simulink model "Taller_1"  (R2025b)
settings: Solver=VariableStepAuto  StartTime=0.0  StopTime=3  RelTol=1e-3
libraries: simulink x8
settings Model: Creator=andre  LastModifiedBy=andre

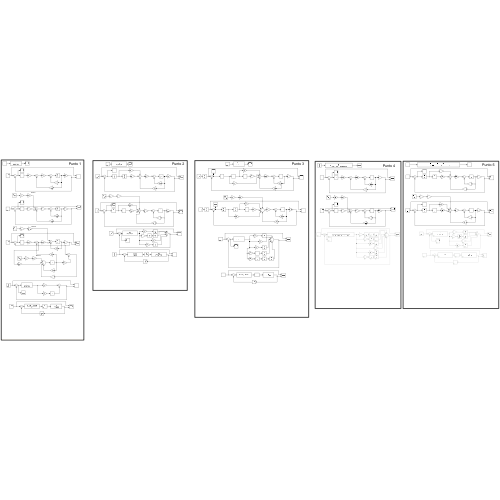
[thumbnail: Simulink's stored preview of the top-level diagram]
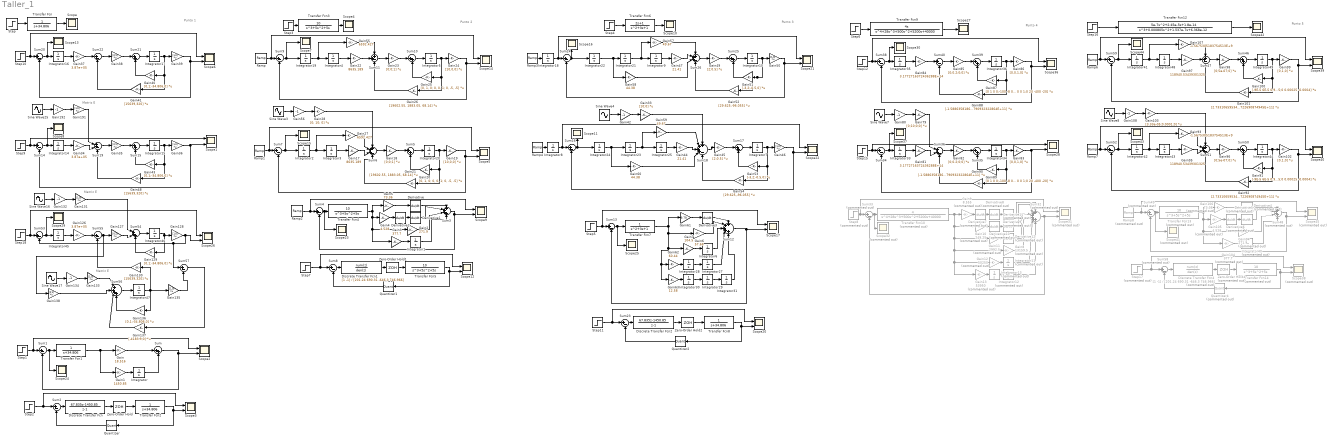
== system Taller_1 ==
  note: Punto 1
  note: Matriz E
  note: Matriz E
  note: Matriz E
  note: Punto 2
  note: Punto 3
  note: Punto 4
  note: Punto 5
  Derivative{,1..3} (4 alike) : Derivative
  Derivative{4..12} (9 alike) : Derivative  Commented=on
  Discrete Transfer Fcn : DiscreteTransferFcn  Numerator=[67.835 -1450.85]  Denominator=[1 -1]
  Discrete Transfer Fcn1 : DiscreteTransferFcn  Numerator=[1 -1]  Denominator=[201.24 690.31 -646.3 746.966]
  Discrete Transfer Fcn2 : DiscreteTransferFcn  Numerator=[67.835 -1450.85]  Denominator=[1 -1]
  Discrete Transfer Fcn4 : DiscreteTransferFcn  Commented=on  Numerator=[1 -1]  Denominator=[201.24 690.31 -646.3 746.966]
  Gain : Gain  Gain=18.516
  Gain1 : Gain  Gain=1450.85
  Gain10 : Gain  Commented=on  Gain=249.25
  Gain100 : Gain  Gain=[-9E-5 6E-5 0;9E-5 -0.000315 0.000125;0 0.00025 -0.0004]  Multiplication=Matrix(K*u)
  Gain101 : Gain  Gain=[2.7331065953402523E+13 282834.44444416161 -2.8927722690874945E+11]  Multiplication=Matrix(K*u)
  Gain102 : Gain  Gain=[0,1,0]  Multiplication=Matrix(K*u)
  Gain103 : Gain  Gain=[3.33e-05;0.0001;0]  Multiplication=Matrix(K*u)
  Gain104 : Gain  Commented=on  Gain=377.7
  Gain105 : Gain  Commented=on  Gain=4.528
  Gain106 : Gain  Commented=on  Gain=73.36
  Gain107 : Gain  Gain=-1.5675305183754513E+9
  Gain{42,56,80,108,132,134,192} (7 alike) : Gain  Gain=-1
  Gain11 : Gain  Commented=on  Gain=2992.5
  Gain12 : Gain  Commented=on  Gain=50250
  Gain126 : Gain  Gain=3.87e+05
  Gain{35,38,127,138} (4 alike) : Gain  Gain=[0;1]  Multiplication=Matrix(K*u)
  Gain{36,39,46,50,128,135} (6 alike) : Gain  Gain=[1,0]  Multiplication=Matrix(K*u)
  Gain{40,43,129,136} (4 alike) : Gain  Gain=[0,1;-34.806,0]  Multiplication=Matrix(K*u)
  Gain13 : Gain  Commented=on  Gain=53950
  Gain130 : Gain  Gain=[15639,320]  Multiplication=Matrix(K*u)
  Gain131 : Gain  Gain=[1;0]  Multiplication=Matrix(K*u)
  Gain133 : Gain  Gain=[1;0]  Multiplication=Matrix(K*u)
  Gain137 : Gain  Gain=[-4183.9;0]  Multiplication=Matrix(K*u)
  Gain17 : Gain  Gain=8635.189
  Gain18 : Gain  Gain=[0;0;1]  Multiplication=Matrix(K*u)
  Gain19 : Gain  Gain=[10,0,0]  Multiplication=Matrix(K*u)
  Gain191 : Gain  Gain=[1;0]  Multiplication=Matrix(K*u)
  Gain2 : Gain  Gain=271.9
  Gain20 : Gain  Gain=[0, 1, 0; 0, 0, 1; 0, -5, -5]  Multiplication=Matrix(K*u)
  Gain21 : Gain  Gain=[19602.55, 1883.05, 68.14]  Multiplication=Matrix(K*u)
  Gain22 : Gain  Gain=8635.189
  Gain23 : Gain  Gain=[0;0;1]  Multiplication=Matrix(K*u)
  Gain24 : Gain  Gain=[10,0,0]  Multiplication=Matrix(K*u)
  Gain25 : Gain  Gain=[0, 1, 0; 0, 0, 1; 0, -5, -5]  Multiplication=Matrix(K*u)
  Gain26 : Gain  Gain=[19602.55, 1883.05, 68.14]  Multiplication=Matrix(K*u)
  Gain27 : Gain  Gain=6592.427
  Gain28 : Gain  Gain=[0; 10; 0]  Multiplication=Matrix(K*u)
  Gain3 : Gain  Gain=377.7
  Gain33 : Gain  Gain=[10;0]  Multiplication=Matrix(K*u)
  Gain34 : Gain  Gain=3.87e+05
  Gain37 : Gain  Gain=3.87e+05
  Gain4 : Gain  Gain=4.528
  Gain41 : Gain  Gain=[15639,320]  Multiplication=Matrix(K*u)
  Gain44 : Gain  Gain=21.41
  Gain45 : Gain  Gain=[2;0.5]  Multiplication=Matrix(K*u)
  Gain47 : Gain  Gain=21.41
  Gain48 : Gain  Gain=[15639,320]  Multiplication=Matrix(K*u)
  Gain49 : Gain  Gain=[2;0.5]  Multiplication=Matrix(K*u)
  Gain5 : Gain  Gain=73.36
  Gain51 : Gain  Gain=[-3,2;-0.5,0]  Multiplication=Matrix(K*u)
  Gain52 : Gain  Gain=[29.625,-96.055]  Multiplication=Matrix(K*u)
  Gain53 : Gain  Gain=[-3,2;-0.5,0]  Multiplication=Matrix(K*u)
  Gain54 : Gain  Gain=[29.625,-96.055]  Multiplication=Matrix(K*u)
  Gain55 : Gain  Gain=6592.427
  Gain57 : Gain  Gain=49.67
  Gain58 : Gain  Gain=44.38
  Gain59 : Gain  Gain=49.67
  Gain6 : Gain  Gain=57.68
  Gain60 : Gain  Gain=44.38
  Gain61 : Gain  Gain=9.79
  Gain62 : Gain  Gain=60.44
  Gain63 : Gain  Gain=12.58
  Gain7 : Gain  Gain=104.5
  Gain79 : Gain  Gain=[0;10;0;0]  Multiplication=Matrix(K*u)
  Gain8 : Gain  Commented=on  Gain=13159.5
  Gain81 : Gain  Gain=3.1772716372436288E+14
  Gain82 : Gain  Gain=[0;0.2;0;0]  Multiplication=Matrix(K*u)
  Gain83 : Gain  Gain=[0,0,1,0]  Multiplication=Matrix(K*u)
  Gain84 : Gain  Gain=3.1772716372436288E+14
  Gain85 : Gain  Gain=[0;0.2;0;0]  Multiplication=Matrix(K*u)
  Gain86 : Gain  Gain=[0,0,1,0]  Multiplication=Matrix(K*u)
  Gain87 : Gain  Gain=[0 1 0 0;-100 -8 0 8;0 0 0 1;0 20 -400 -20]  Multiplication=Matrix(K*u)
  Gain88 : Gain  Gain=[-1.5886358186321061E+13 67.6956684856248 1.5886358185456043E+13 7.9431790932322864E+11]  Multiplication=Matrix(K*u)
  Gain89 : Gain  Gain=[0 1 0 0;-100 -8 0 8;0 0 0 1;0 20 -400 -20]  Multiplication=Matrix(K*u)
  Gain9 : Gain  Commented=on  Gain=8.555
  Gain90 : Gain  Gain=[-1.5886358186321061E+13 67.6956684856248 1.5886358185456043E+13 7.9431790932322864E+11]  Multiplication=Matrix(K*u)
  Gain91 : Gain  Gain=[-9E-5 6E-5 0;9E-5 -0.000315 0.000125;0 0.00025 -0.0004]  Multiplication=Matrix(K*u)
  Gain92 : Gain  Gain=[2.7331065953402523E+13 282834.44444416161 -2.8927722690874945E+11]  Multiplication=Matrix(K*u)
  Gain93 : Gain  Gain=-1.5675305183754513E+9
  Gain94 : Gain  Commented=on  Gain=271.9
  Gain95 : Gain  Gain=118940.53439301325
  Gain96 : Gain  Gain=[0;5e-07;0]  Multiplication=Matrix(K*u)
  Gain97 : Gain  Gain=118940.53439301325
  Gain98 : Gain  Gain=[0;5e-07;0]  Multiplication=Matrix(K*u)
  Gain99 : Gain  Gain=[0,1,0]  Multiplication=Matrix(K*u)
  Integrator{,1..10,14..25,27..31,33..36,41..49} (41 alike) : Integrator
  Integrator{11..13,40} (4 alike) : Integrator  Commented=on
  Quantizer : Quantizer  QuantizationInterval=3.3/1024
  Quantizer1 : Quantizer  QuantizationInterval=3.3/1024
  Quantizer2 : Quantizer  QuantizationInterval=3.3/1024
  Quantizer4 : Quantizer  Commented=on  QuantizationInterval=3.3/1024
  Ramp{,1..4,6..7} (7 alike) : simulink/Sources/Ramp  slope=1  start=0  InitialOutput=0
  Ramp8 : simulink/Sources/Ramp  Commented=on  slope=1  start=0  InitialOutput=0
  Scope{,4,7..8,10..11,13,15..16,23..25,27,29..30,37,42..44} (19 alike) : Scope
      Scope settings: ActiveDisplayYMinimum=-0.0071982318273006371  ActiveDisplayYMaximum=0.031818468747388327
      Scope10 settings: ActiveDisplayYMinimum=-0.12488775902717804  ActiveDisplayYMaximum=1.1239898312446026  DataLoggingVariableName=ScopeData3
      Scope11 settings: ActiveDisplayYMinimum=-1  ActiveDisplayYMaximum=1  DataLoggingVariableName=ScopeData4
      Scope13 settings: ActiveDisplayYMinimum=-1  ActiveDisplayYMaximum=1  DataLoggingVariableName=ScopeData12
      Scope15 settings: ActiveDisplayYMinimum=-0.033671475717911077  ActiveDisplayYMaximum=0.27729553793845596  DataLoggingVariableName=ScopeData10
      Scope16 settings: ActiveDisplayYMinimum=-1  ActiveDisplayYMaximum=1  DataLoggingVariableName=ScopeData16
      Scope23 settings: DataLoggingVariableName=ScopeData23
      Scope24 settings: DataLoggingVariableName=ScopeData24
      Scope25 settings: ActiveDisplayYMinimum=-0.36214218319670444  ActiveDisplayYMaximum=1.1513491314663005  DataLoggingVariableName=ScopeData26
      Scope27 settings: ActiveDisplayYMinimum=-0.00057991321568763013  ActiveDisplayYMaximum=0.00092074928311051279  DataLoggingVariableName=ScopeData27
      Scope29 settings: ActiveDisplayYMinimum=-0.003476814901466117  ActiveDisplayYMaximum=0.031291334113195061  DataLoggingVariableName=ScopeData28
      Scope30 settings: ActiveDisplayYMinimum=-1  ActiveDisplayYMaximum=1  DataLoggingVariableName=ScopeData30
      Scope37 settings: ActiveDisplayYMinimum=-1  ActiveDisplayYMaximum=1  DataLoggingVariableName=ScopeData37
      Scope4 settings: ActiveDisplayYMinimum=-0.26842236879798326  ActiveDisplayYMaximum=2.41580131918185  DataLoggingVariableName=ScopeData11
      Scope42 settings: ActiveDisplayYMinimum=-0.33520594716495827  ActiveDisplayYMaximum=3.0168535244846248  DataLoggingVariableName=ScopeData42
      Scope43 settings: ActiveDisplayYMinimum=-1.9029513689588776E+6  ActiveDisplayYMaximum=5.5810175747817233E+6  DataLoggingVariableName=ScopeData43
      Scope44 settings: ActiveDisplayYMinimum=-1  ActiveDisplayYMaximum=1  DataLoggingVariableName=ScopeData44
      Scope7 settings: ActiveDisplayYMinimum=-1  ActiveDisplayYMaximum=1  DataLoggingVariableName=ScopeData14
      Scope8 settings: ActiveDisplayYMinimum=-1  ActiveDisplayYMaximum=1  DataLoggingVariableName=ScopeData7
  Scope{1..3,5..6,9,12,14,17,20..22,26,28,36,39..40} (17 alike) : Scope  NumInputPorts=2
      Scope1 settings: ActiveDisplayYMinimum=-0.13055074104644734  ActiveDisplayYMaximum=1.1749566694180262  DataLoggingVariableName=ScopeData5
      Scope12 settings: ActiveDisplayYMinimum=-3.48363499121058E+35  ActiveDisplayYMaximum=1.1703123918708805E+35  DataLoggingVariableName=ScopeData6
      Scope14 settings: ActiveDisplayYMinimum=-0.62499999999999989  ActiveDisplayYMaximum=5.625  DataLoggingVariableName=ScopeData8
      Scope17 settings: ActiveDisplayYMinimum=-0.15134913146630047  ActiveDisplayYMaximum=1.3621421831967044  DataLoggingVariableName=ScopeData17
      Scope2 settings: ActiveDisplayYMinimum=-0.13187455988119548  ActiveDisplayYMaximum=1.1868710389307595
      Scope20 settings: ActiveDisplayYMinimum=-1  ActiveDisplayYMaximum=1  DataLoggingVariableName=ScopeData20
      Scope21 settings: ActiveDisplayYMinimum=-1.0198271839956574  ActiveDisplayYMaximum=9.1784446559609183  DataLoggingVariableName=ScopeData21
      Scope22 settings: ActiveDisplayYMinimum=-14.062552935850418  ActiveDisplayYMaximum=126.56297642265379  DataLoggingVariableName=ScopeData22
      Scope26 settings: ActiveDisplayYMinimum=-1  ActiveDisplayYMaximum=1  DataLoggingVariableName=ScopeData25
      Scope28 settings: ActiveDisplayYMinimum=-5.245661607857852E+9  ActiveDisplayYMaximum=4.7210954470720673E+10  DataLoggingVariableName=ScopeData29
      Scope3 settings: ActiveDisplayYMinimum=-1  ActiveDisplayYMaximum=1  DataLoggingVariableName=ScopeData2
      Scope36 settings: ActiveDisplayYMinimum=-5.24563506830911E+9  ActiveDisplayYMaximum=4.7210715614782E+10  DataLoggingVariableName=ScopeData36
      Scope39 settings: ActiveDisplayYMinimum=-8165.2546159211288  ActiveDisplayYMaximum=911.6949573245696  DataLoggingVariableName=ScopeData39
      Scope40 settings: ActiveDisplayYMinimum=-5.63952560953284E+6  ActiveDisplayYMaximum=1.9129703378474237E+6  DataLoggingVariableName=ScopeData40
      Scope5 settings: ActiveDisplayYMinimum=-0.62499999999999989  ActiveDisplayYMaximum=5.625  DataLoggingVariableName=ScopeData13
      Scope6 settings: ActiveDisplayYMinimum=-0.13068042045208161  ActiveDisplayYMaximum=1.1761237840687349  DataLoggingVariableName=ScopeData9
      Scope9 settings: ActiveDisplayYMinimum=-1.2500000000852405  ActiveDisplayYMaximum=11.250000000009472  DataLoggingVariableName=ScopeData15
  Scope31 : Scope  Commented=on  NumInputPorts=2
      settings: ActiveDisplayYMinimum=-0.13187455988119548  ActiveDisplayYMaximum=1.1868710389307595  DataLoggingVariableName=ScopeData31
  Scope32 : Scope  Commented=on
      settings: DataLoggingVariableName=ScopeData32
  Scope38 : Scope  Commented=on  NumInputPorts=2
      settings: ActiveDisplayYMinimum=-3.48363499121058E+35  ActiveDisplayYMaximum=1.1703123918708805E+35  DataLoggingVariableName=ScopeData38
  Scope41 : Scope  Commented=on
      settings: DataLoggingVariableName=ScopeData41
  Scope45 : Scope  Commented=on  NumInputPorts=2
      settings: ActiveDisplayYMinimum=-1.2500000000852405  ActiveDisplayYMaximum=11.250000000009472  DataLoggingVariableName=ScopeData45
  Sine Wave{3..4,7..8,16..17,25} (7 alike) : Sin  SampleTime=0
  Step{,1..7,9..12,15..16,18} (15 alike) : Step  Time=0  SampleTime=0
  Step17 : Step  Commented=on  Time=0  SampleTime=0
  Step8 : Step  Commented=on  Time=0  SampleTime=0
  Sum{,5,10,15,17,21,25,35,39,46,50} (11 alike) : Sum  Inputs=|++
  Sum{1..2,4,7..9,13..14,16,20,22..24,34,38,40,52..53,55,57,59} (21 alike) : Sum  Inputs=|+-
  Sum11 : Sum  Inputs=++-
  Sum12 : Sum  Inputs=+++++
  Sum18 : Sum  Inputs=++++-
  Sum19 : Sum  Inputs=|++-
  Sum26 : Sum  Inputs=+++-
  Sum3 : Sum  Inputs=++++
  Sum32 : Sum  Commented=on  Inputs=++++++
  Sum33 : Sum  Commented=on  Inputs=|+-
  Sum36 : Sum  Inputs=|++-
  Sum47 : Sum  Inputs=++-
  Sum48 : Sum  Commented=on  Inputs=++++
  Sum49 : Sum  Commented=on  Inputs=|+-
  Sum51 : Sum  Inputs=+++-
  Sum54 : Sum  Inputs=|+++
  Sum56 : Sum  Inputs=|++++
  Sum58 : Sum  Commented=on  Inputs=|+-
  Sum6 : Sum  Inputs=+++-
  Transfer Fcn{,1..2,8} (4 alike) : TransferFcn  Denominator=[1 34.806]
  Transfer Fcn10 : TransferFcn  Commented=on  Numerator=[4]  Denominator=[1 28 500 5200 40000]
  Transfer Fcn12 : TransferFcn  Numerator=[5e-7 2.45e-5 1.8e-14]  Denominator=[1 0.000805 1.537e-7 6.368e-12]
  Transfer Fcn13 : TransferFcn  Commented=on  Numerator=[10]  Denominator=[1 5 5 0]
  Transfer Fcn14 : TransferFcn  Commented=on  Numerator=[10]  Denominator=[1 5 5 0]
  Transfer Fcn3 : TransferFcn  Numerator=[10]  Denominator=[1 5 5 0]
  Transfer Fcn4 : TransferFcn  Numerator=[10]  Denominator=[1 5 5 0]
  Transfer Fcn5 : TransferFcn  Numerator=[10]  Denominator=[1 5 5 0]
  Transfer Fcn6 : TransferFcn  Numerator=[2 1]  Denominator=[1 3 1]
  Transfer Fcn7 : TransferFcn  Denominator=[1 3 1]
  Transfer Fcn9 : TransferFcn  Numerator=[4 0]  Denominator=[1 28 500 5200 40000]
  Zero-Order Hold : ZeroOrderHold  SampleTime=0.01
  Zero-Order Hold1 : ZeroOrderHold  SampleTime=0.15
  Zero-Order Hold2 : ZeroOrderHold  SampleTime=0.01
  Zero-Order Hold4 : ZeroOrderHold  Commented=on  SampleTime=0.15
  wires:
  Step/1 -> Transfer Fcn/1
  Transfer Fcn/1 -> Scope/1
  Gain41/1 -> Sum22/2
  Integrator15/1 -> Gain36/1, Gain43/1, Gain48/1
  Sum19/1 -> Gain35/1
  Gain39/1 -> Scope6/2, Sum20/2
  Sum22/1 -> Gain38/1
  Sine Wave25/1 -> Gain192/1
  Sum14/1 -> Scope8/1, Integrator14/1
  Gain43/1 -> Sum15/2
  Gain48/1 -> Sum19/3
  Step9/1 -> Scope1/1, Sum14/1
  Gain192/1 -> Gain191/1
  Step10/1 -> Scope6/1, Sum20/1
  Sum21/1 -> Integrator17/1
  Sum15/1 -> Integrator15/1
  Gain37/1 -> Sum22/1
  Gain36/1 -> Sum14/2, Scope1/2
  Gain40/1 -> Sum21/2
  Gain191/1 -> Sum19/1
  Integrator17/1 -> Gain41/1, Gain40/1, Gain39/1
  Integrator16/1 -> Gain37/1
  Gain34/1 -> Sum19/2
  Sum20/1 -> Scope13/1, Integrator16/1
  Gain35/1 -> Sum15/1
  Integrator14/1 -> Gain34/1
  Gain38/1 -> Sum21/1
  Sine Wave16/1 -> Gain132/1
  Gain128/1 -> Scope26/2, Sum57/1, Sum53/2
  Integrator45/1 -> Gain126/1
  Gain127/1 -> Sum54/2
  Gain136/1 -> Sum56/4
  Sum57/1 -> Gain137/1
  Sine Wave17/1 -> Gain134/1
  Gain132/1 -> Gain131/1
  Gain130/1 -> Sum55/2
  Integrator47/1 -> Gain135/1, Gain136/1, Gain130/1
  Gain134/1 -> Gain133/1
  Gain133/1 -> Sum56/1
  Sum53/1 -> Scope29/1, Integrator45/1
  Sum56/1 -> Integrator47/1
  Integrator46/1 -> Gain129/1, Gain128/1
  Gain137/1 -> Sum56/3
  Gain129/1 -> Sum54/3
  Gain135/1 -> Sum57/2
  Gain131/1 -> Sum54/1
  Step18/1 -> Scope26/1, Sum53/1
  Gain138/1 -> Sum56/2
  Sum54/1 -> Integrator46/1
  Gain126/1 -> Sum55/1
  Sum55/1 -> Gain127/1, Gain138/1
  Gain1/1 -> Integrator/1
  Gain/1 -> Sum/1
  Integrator/1 -> Sum/2
  Sum/1 -> Sum1/2, Scope2/2
  Transfer Fcn1/1 -> Gain1/1, Gain/1
  Sum1/1 -> Scope24/1, Transfer Fcn1/1
  Step1/1 -> Sum1/1, Scope2/1
  Zero-Order Hold/1 -> Transfer Fcn2/1
  Quantizer/1 -> Sum2/2
  Transfer Fcn2/1 -> Scope3/2, Quantizer/1
  Sum2/1 -> Discrete Transfer Fcn/1
  Discrete Transfer Fcn/1 -> Zero-Order Hold/1
  Step2/1 -> Sum2/1, Scope3/1
  Discrete Transfer Fcn1/1 -> Zero-Order Hold1/1
  Ramp2/1 -> Sum4/1, Scope9/1
  Sum4/1 -> Scope23/1, Transfer Fcn4/1
  Sum8/1 -> Discrete Transfer Fcn1/1
  Gain2/1 -> Sum3/3
  Sum9/1 -> Integrator19/1, Scope7/1
  Integrator4/1 -> Gain22/1
  Quantizer1/1 -> Sum8/2
  Gain22/1 -> Sum11/2
  Integrator5/1 -> Gain26/1, Gain25/1, Gain24/1
  Zero-Order Hold1/1 -> Transfer Fcn5/1
  Gain23/1 -> Sum10/1
  Step7/1 -> Sum8/1, Scope12/1
  Gain25/1 -> Sum10/2
  Sum11/1 -> Gain23/1
  Gain24/1 -> Scope14/2, Sum9/2
  Gain26/1 -> Sum11/3
  Sum10/1 -> Integrator5/1
  Transfer Fcn5/1 -> Scope12/2, Quantizer1/1
  Integrator1/1 -> Sum3/4
  Transfer Fcn4/1 -> Gain4/1, Gain2/1, Gain3/1, Gain5/1
  Sum3/1 -> Sum4/2, Scope9/2
  Transfer Fcn3/1 -> Scope4/1
  Gain3/1 -> Integrator1/1
  Ramp/1 -> Scope14/1, Sum9/1
  Step3/1 -> Transfer Fcn3/1
  Derivative2/1 -> Derivative1/1
  Gain4/1 -> Derivative2/1
  Gain5/1 -> Derivative/1
  Derivative/1 -> Sum3/1
  Derivative1/1 -> Sum3/2
  Integrator9/1 -> Gain47/1
  Step11/1 -> Sum23/1, Scope20/1
  Gain51/1 -> Sum25/2
  Sum23/1 -> Discrete Transfer Fcn2/1
  Transfer Fcn6/1 -> Scope10/1
  Sum12/1 -> Sum13/2, Scope17/2
  Sum25/1 -> Integrator10/1
  Gain7/1 -> Integrator6/1
  Step5/1 -> Sum13/1, Scope17/1
  Gain50/1 -> Scope21/2, Sum24/2
  Integrator10/1 -> Gain52/1, Gain51/1, Gain50/1
  Sum13/1 -> Scope25/1, Transfer Fcn7/1
  Gain42/1 -> Gain33/1
  Integrator18/1 -> Sum24/1, Scope21/1
  Transfer Fcn7/1 -> Gain61/1, Gain63/1, Gain62/1, Gain7/1, Gain6/1
  Sum26/1 -> Gain49/1
  Step4/1 -> Transfer Fcn6/1
  Sum24/1 -> Integrator22/1, Scope16/1
  Sine Wave4/1 -> Gain42/1
  Zero-Order Hold2/1 -> Transfer Fcn8/1
  Gain47/1 -> Sum26/2
  Quantizer2/1 -> Sum23/2
  Discrete Transfer Fcn2/1 -> Zero-Order Hold2/1
  Gain52/1 -> Sum26/4
  Gain49/1 -> Sum25/1
  Transfer Fcn8/1 -> Scope20/2, Quantizer2/1
  Ramp3/1 -> Integrator18/1
  Integrator19/1 -> Gain55/1, Integrator4/1
  Gain55/1 -> Sum11/1
  Gain21/1 -> Sum6/4
  Gain17/1 -> Sum6/3
  Gain27/1 -> Sum6/2
  Gain18/1 -> Sum5/1
  Sum5/1 -> Integrator20/1
  Integrator3/1 -> Gain17/1
  Ramp1/1 -> Scope5/1, Sum7/1
  Sum7/1 -> Integrator2/1, Scope15/1
  Sum6/1 -> Gain18/1
  Gain20/1 -> Sum5/2
  Gain19/1 -> Scope5/2, Sum7/2
  Integrator2/1 -> Gain27/1, Integrator3/1
  Integrator20/1 -> Gain21/1, Gain20/1, Gain19/1
  Sine Wave3/1 -> Gain56/1
  Gain56/1 -> Gain28/1
  Gain28/1 -> Sum6/1
  Integrator21/1 -> Gain57/1, Integrator9/1
  Integrator22/1 -> Gain58/1, Integrator21/1
  Gain58/1 -> Sum26/3
  Gain57/1 -> Sum26/1
  Gain59/1 -> Sum18/2
  Gain44/1 -> Sum18/3
  Integrator24/1 -> Gain60/1, Integrator23/1
  Ramp4/1 -> Integrator8/1
  Gain45/1 -> Sum17/1
  Sum16/1 -> Integrator24/1, Scope11/1
  Sum18/1 -> Gain45/1
  Integrator7/1 -> Gain54/1, Gain53/1, Gain46/1
  Integrator8/1 -> Sum16/1, Scope22/1
  Integrator25/1 -> Gain44/1
  Gain53/1 -> Sum17/2
  Gain46/1 -> Scope22/2, Sum16/2
  Gain54/1 -> Sum18/5
  Integrator23/1 -> Gain59/1, Integrator25/1
  Gain60/1 -> Sum18/4
  Sum17/1 -> Integrator7/1
  Gain33/1 -> Sum18/1
  Gain61/1 -> Derivative3/1
  Integrator29/1 -> Integrator31/1
  Integrator28/1 -> Integrator27/1
  Integrator30/1 -> Integrator29/1
  Gain62/1 -> Integrator28/1
  Gain63/1 -> Integrator30/1
  Derivative3/1 -> Sum12/1
  Gain6/1 -> Sum12/2
  Integrator6/1 -> Sum12/3
  Integrator27/1 -> Sum12/4
  Integrator31/1 -> Sum12/5
  Integrator35/1 -> Gain84/1
  Gain82/1 -> Sum35/1
  Sum36/1 -> Gain82/1
  Gain87/1 -> Sum39/2
  Integrator34/1 -> Gain83/1, Gain89/1, Gain90/1
  Transfer Fcn9/1 -> Scope27/1
  Sum32/1 -> Sum33/2, Scope31/2
  Gain90/1 -> Sum36/3
  Sum39/1 -> Integrator36/1
  Gain81/1 -> Sum36/2
  Step15/1 -> Scope28/1, Sum34/1
  Gain89/1 -> Sum35/2
  Step8/1 -> Sum33/1, Scope31/1
  Gain79/1 -> Sum36/1
  Gain83/1 -> Sum34/2, Scope28/2
  Gain86/1 -> Scope36/2, Sum38/2
  Integrator36/1 -> Gain88/1, Gain87/1, Gain86/1
  Sum33/1 -> Scope32/1, Transfer Fcn10/1
  Gain80/1 -> Gain79/1
  Integrator33/1 -> Gain81/1
  Step12/1 -> Scope36/1, Sum38/1
  Sum40/1 -> Gain85/1
  Step6/1 -> Transfer Fcn9/1
  Sum35/1 -> Integrator34/1
  Sum38/1 -> Scope30/1, Integrator35/1
  Sine Wave7/1 -> Gain80/1
  Sum34/1 -> Scope37/1, Integrator33/1
  Gain84/1 -> Sum40/1
  Gain88/1 -> Sum40/2
  Gain85/1 -> Sum39/1
  Sum58/1 -> Discrete Transfer Fcn4/1
  Zero-Order Hold4/1 -> Transfer Fcn14/1
  Ramp6/1 -> Scope39/1, Sum59/1
  Integrator41/1 -> Gain107/1, Integrator48/1
  Step16/1 -> Transfer Fcn12/1
  Gain99/1 -> Scope39/2, Sum59/2
  Gain105/1 -> Derivative6/1
  Ramp8/1 -> Sum49/1, Scope45/1
  Gain100/1 -> Sum46/2
  Derivative5/1 -> Sum48/2
  Gain94/1 -> Sum48/3
  Discrete Transfer Fcn4/1 -> Zero-Order Hold4/1
  Transfer Fcn14/1 -> Scope38/2, Quantizer4/1
  Quantizer4/1 -> Sum58/2
  Sine Wave8/1 -> Gain108/1
  Transfer Fcn13/1 -> Gain105/1, Gain94/1, Gain104/1, Gain106/1
  Gain104/1 -> Integrator40/1
  Gain108/1 -> Gain103/1
  Sum59/1 -> Integrator41/1, Scope44/1
  Derivative6/1 -> Derivative5/1
  Gain106/1 -> Derivative4/1
  Sum48/1 -> Sum49/2, Scope45/2
  Integrator49/1 -> Gain101/1, Gain100/1, Gain99/1
  Step17/1 -> Sum58/1, Scope38/1
  Transfer Fcn12/1 -> Scope42/1
  Gain98/1 -> Sum46/1
  Sum47/1 -> Gain98/1
  Sum49/1 -> Scope41/1, Transfer Fcn13/1
  Gain97/1 -> Sum47/2
  Gain107/1 -> Sum47/1
  Integrator40/1 -> Sum48/4
  Integrator48/1 -> Gain97/1
  Gain101/1 -> Sum47/3
  Derivative4/1 -> Sum48/1
  Sum46/1 -> Integrator49/1
  Ramp7/1 -> Scope40/1, Sum52/1
  Integrator44/1 -> Gain92/1, Gain91/1, Gain102/1
  Sum52/1 -> Integrator42/1, Scope43/1
  Gain102/1 -> Scope40/2, Sum52/2
  Gain91/1 -> Sum50/2
  Integrator43/1 -> Gain95/1
  Gain95/1 -> Sum51/3
  Gain93/1 -> Sum51/2
  Gain96/1 -> Sum50/1
  Sum51/1 -> Gain96/1
  Integrator42/1 -> Gain93/1, Integrator43/1
  Sum50/1 -> Integrator44/1
  Gain92/1 -> Sum51/4
  Gain103/1 -> Sum51/1
  Derivative7/1 -> Derivative8/1
  Derivative8/1 -> Derivative9/1
  Derivative10/1 -> Derivative11/1
  Integrator13/1 -> Integrator12/1
  Gain9/1 -> Derivative7/1
  Gain10/1 -> Derivative10/1
  Gain11/1 -> Derivative12/1
  Gain12/1 -> Integrator11/1
  Gain13/1 -> Integrator13/1
  Transfer Fcn10/1 -> Gain13/1, Gain12/1, Gain8/1, Gain11/1, Gain10/1, Gain9/1
  Derivative9/1 -> Sum32/1
  Derivative11/1 -> Sum32/2
  Derivative12/1 -> Sum32/3
  Gain8/1 -> Sum32/4
  Integrator11/1 -> Sum32/5
  Integrator12/1 -> Sum32/6
